simulink model "EE382lab53"  (R2016a)
settings: Solver=VariableStepAuto  StartTime=0.0  StopTime=1.0  RelTol=1e-3
libraries: dsparch4 x2
settings Model: Creator=Tryrant  LastModifiedBy=Tryrant

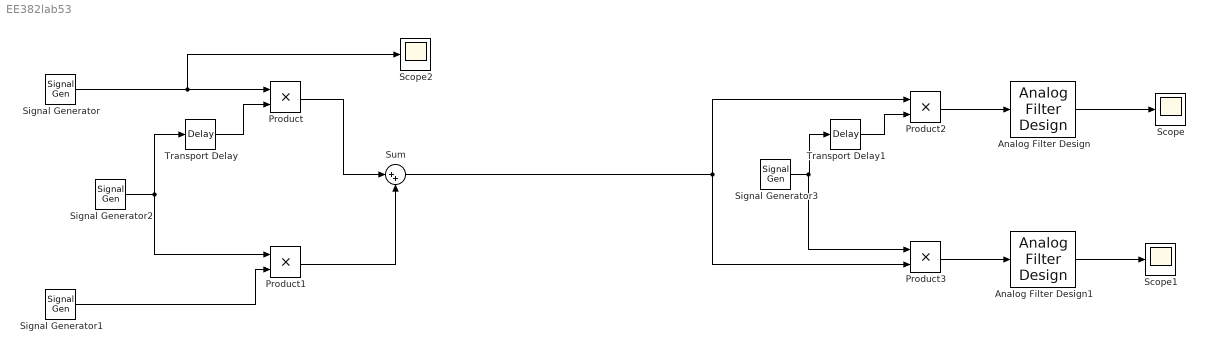
== system EE382lab53 ==
  Analog Filter Design : dsparch4/Analog Filter Design  method=Butterworth  filttype=Lowpass  N=8  Wlo=2*pi*800*2  Whi=80  Rp=2  Rs=40
  Analog Filter Design1 : dsparch4/Analog Filter Design  method=Butterworth  filttype=Lowpass  N=8  Wlo=2000*2*pi*2  Whi=80  Rp=2  Rs=40
  Product{,1..3} (4 alike) : Product
  Scope : Scope
  Scope1 : Scope
  Scope2 : Scope
  Signal Generator : SignalGenerator  Amplitude=3  Frequency=800
  Signal Generator1 : SignalGenerator  Amplitude=10  Frequency=2000
  Signal Generator2 : SignalGenerator  Frequency=300000
  Signal Generator3 : SignalGenerator  Amplitude=2  Frequency=300000
  Sum : Sum  Inputs=|++
  Transport Delay : TransportDelay  DelayTime=1/(4*300000)  BufferSize=4026
  Transport Delay1 : TransportDelay  DelayTime=1/(4*300000)  BufferSize=4026
  wires:
  Signal Generator/1 -> Scope2/1, Product/1
  Signal Generator1/1 -> Product1/2
  Product/1 -> Sum/1
  Product1/1 -> Sum/2
  Sum/1 -> Product2/1, Product3/2
  Product3/1 -> Analog Filter Design1/1
  Analog Filter Design1/1 -> Scope1/1
  Transport Delay/1 -> Product/2
  Signal Generator2/1 -> Product1/1, Transport Delay/1
  Transport Delay1/1 -> Product2/2
  Signal Generator3/1 -> Product3/1, Transport Delay1/1
  Product2/1 -> Analog Filter Design/1
  Analog Filter Design/1 -> Scope/1
